simulink subsystem "sistema_nonlineare"  (R2019b)
settings: Solver=VariableStepAuto  StartTime=0.0  StopTime=10.0  RelTol=1e-3
values from neighbouring files (symbols this model uses):
  tab_a_inv = 1/(pi^2)    (= 0.101321183642)    [progetto_3A.m]
  tab_C_d = 2*pi^2    (= 19.7392088022)    [progetto_3A.m]
  tab_eta = 0.6    [progetto_3A.m]
  tab_g_const = 9.80655    [progetto_3A.m]
  tab_R_0 = 45    [progetto_3A.m]
  tab_x_equilibrio_1 = 10    [progetto_3A.m]
  tab_x_equilibrio_2 = 6    [progetto_3A.m]
  tab_x_equilibrio_3 = 6    [progetto_3A.m]
settings Model: Creator=Luca  LastModifiedBy=Luca

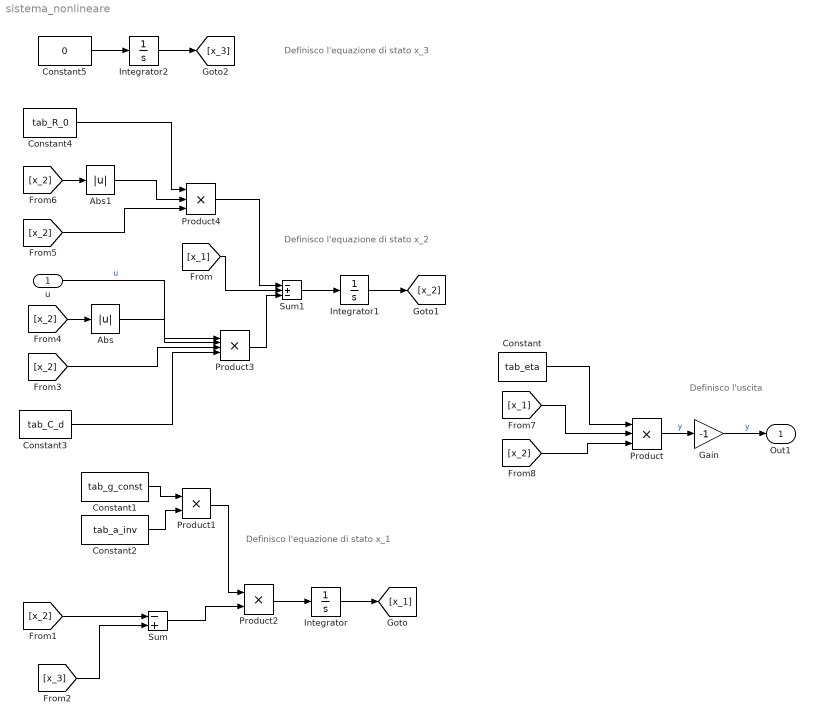
== system sistema_nonlineare ==
  note: Definisco l'uscita
  note: Definisco l'equazione di stato x_1
  note: Definisco l'equazione di stato x_2
  note: Definisco l'equazione di stato x_3
  u : Inport
  Abs : Abs
  Abs1 : Abs
  Constant : Constant  Value=tab_eta
  Constant1 : Constant  Value=tab_g_const
  Constant2 : Constant  Value=tab_a_inv
  Constant3 : Constant  Value=tab_C_d
  Constant4 : Constant  Value=tab_R_0
  Constant5 : Constant  Value=0
  Gain : Gain  Gain=-1
  Integrator : Integrator  InitialCondition=tab_x_equilibrio_1
  Integrator1 : Integrator  InitialCondition=tab_x_equilibrio_2
  Integrator2 : Integrator  InitialCondition=tab_x_equilibrio_3
  Product : Product  Inputs=3
  Product1 : Product
  Product2 : Product
  Product3 : Product  Inputs=4
  Product4 : Product  Inputs=3
  Sum : Sum  Inputs=-+
  Sum1 : Sum  Inputs=-+-
  Out1 : Outport
  wires:
  Constant/1 -> Product/1
  Constant1/1 -> Product1/1
  [x_3] -> Sum/2
  Product1/1 -> Product2/1
  Sum/1 -> Product2/2
  Product2/1 -> Integrator/1
  Integrator/1 -> [x_1]
  [x_2] -> Abs/1
  u/1 -> Product3/1  "u"
  Abs/1 -> Product3/2
  [x_2] -> Product3/3
  [x_2] -> Abs1/1
  [x_2] -> Product4/3
  Abs1/1 -> Product4/2
  Constant4/1 -> Product4/1
  Product4/1 -> Sum1/1
  [x_1] -> Sum1/2
  Integrator1/1 -> [x_2]
  Sum1/1 -> Integrator1/1
  Integrator2/1 -> [x_3]
  Constant5/1 -> Integrator2/1
  [x_1] -> Product/2
  [x_2] -> Product/3
  Constant2/1 -> Product1/2
  [x_2] -> Sum/1
  Product/1 -> Gain/1  "y"
  Gain/1 -> Out1/1  "y"
  Product3/1 -> Sum1/3
  Constant3/1 -> Product3/4
